simulink model "water_tank"  (R2024b)
settings: Solver=VariableStepAuto  StartTime=0.0  StopTime=inf  RelTol=1e-3
settings Model: Creator=HP  LastModifiedBy=HP

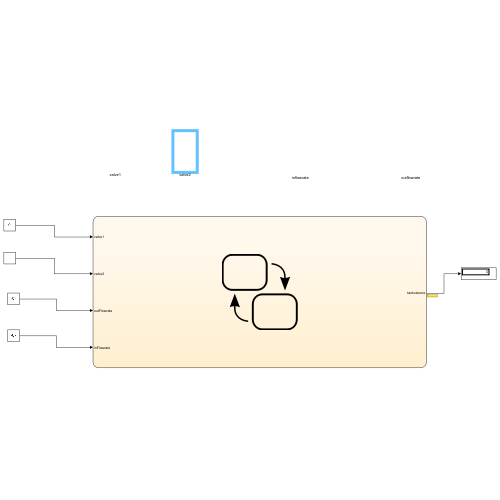
[thumbnail: Simulink's stored preview of the top-level diagram]
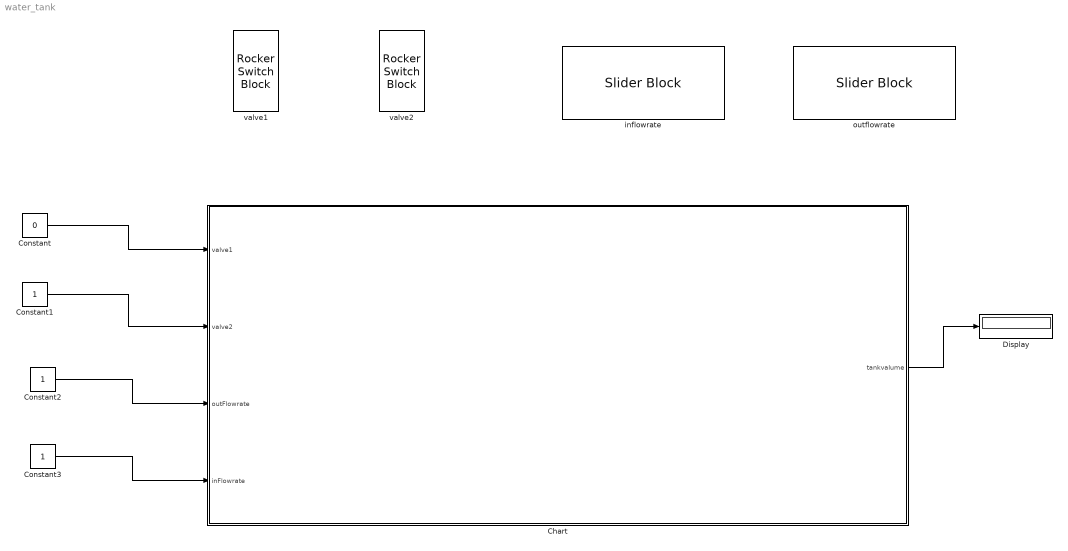
== system water_tank ==
  Chart : Stateflow chart  TreatAsAtomicUnit=on
  Constant : Constant  Value=0
  Constant1 : Constant
  Constant2 : Constant
  Constant3 : Constant
  Display : Display
  inflowrate : SliderBlock  ScaleMax=1
  outflowrate : SliderBlock  ScaleMax=1
  valve1 : RockerSwitchBlock
      settings: Values={{'Off', 'On'}, [0 1]}
  valve2 : RockerSwitchBlock
      settings: Values={{'Off', 'On'}, [0 1]}
  wires:
  Constant/1 -> Chart/1(valve1)
  Constant1/1 -> Chart/2(valve2)
  Constant2/1 -> Chart/3(outFlowrate)
  Constant3/1 -> Chart/4(inFlowrate)
  Chart/1(tankvalume) -> Display/1

== stateflow chart water_tank/Chart ==
  state water_tank
    state fill [parallel]
      settings: executionOrder=1
      state valve1_close
      state valve1_open
        tankvalume=min((tankvalume+inFlowrate),100);
      (default) -> valve1_close
      valve1_close -> valve1_open : [valve1==1&&...
          | tankvalume<=100]
      valve1_open -> valve1_close : [valve1==0||...
          | tankvalume>=100]
    state empty [parallel]
      settings: executionOrder=2
      state valve2_close
      state valve2_open
        tankvalume=max((tankvalume-outFlowrate), 0);
      (default) -> valve2_close
      valve2_close -> valve2_open : [valve2==1&&...
          | tankvalume>=0]
      valve2_open -> valve2_close : [valve2==0||...
          | tankvalume<=0]
    (default) -> empty
  (default) -> water_tank
  data: valve1 input; valve2 input; outFlowrate input; inFlowrate input; tankvalume output [0..100] =0
